simulink model "Delta_Sigma_ADC_Deg3"  (R2025b)
settings: Solver=VariableStepAuto  StartTime=0.0  StopTime=15  RelTol=1e-3
undefined symbols (not defined in the file): DiscIntNeverNeededParam
settings Model: Creator=Yash  LastModifiedBy=Yash
settings DataIOCC: SaveOutput=off  SaveTime=off
settings HardwareCC: ProdBitPerPointer=32.0  ProdBitPerSizeT=32.0  ProdBitPerPtrDiffT=32.0  ProdLargestAtomicFloat=None  ProdIntDivRoundTo=Undefined  ProdEndianess=Unspecified  ProdWordSize=32.0  ProdHWDeviceType=ASIC/FPGA->ASIC/FPGA  TargetBitPerPointer=64.0  TargetBitPerSizeT=64.0  TargetBitPerPtrDiffT=64.0  TargetLongLongMode=on  TargetIntDivRoundTo=Zero  TargetEndianess=LittleEndian  TargetWordSize=64.0  TargetHWDeviceType=Custom Processor->MATLAB Host Computer  ProdEqTarget=off

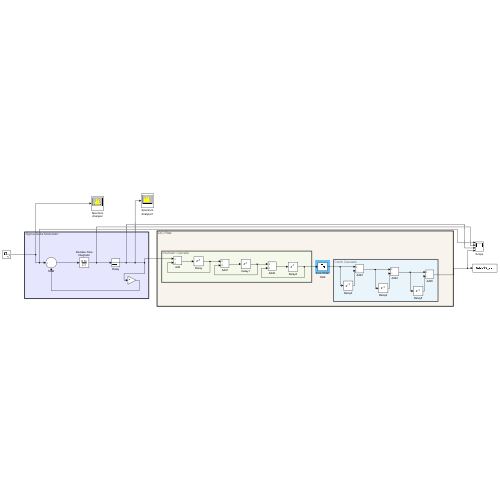
[thumbnail: Simulink's stored preview of the top-level diagram]
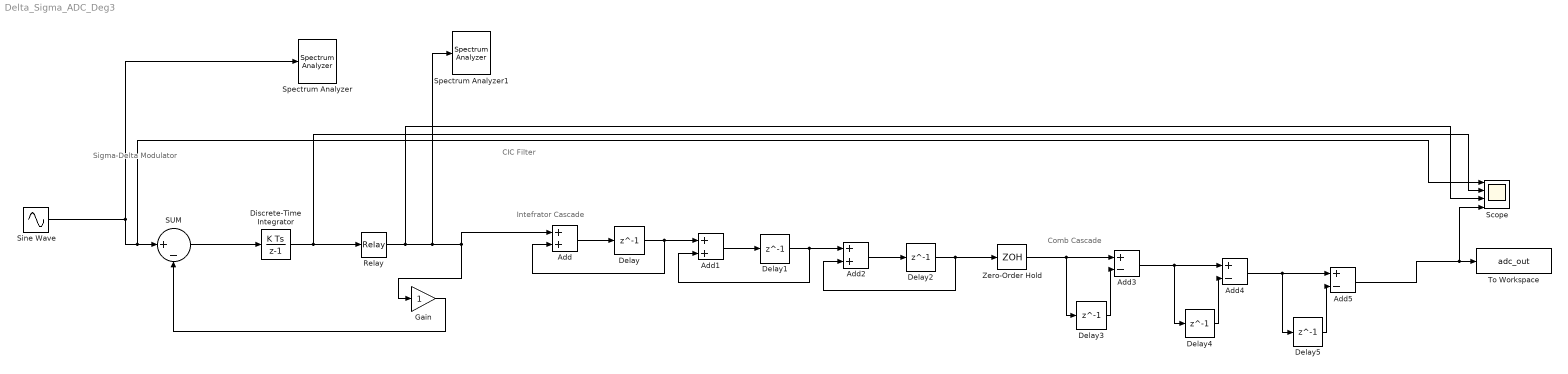
== system Delta_Sigma_ADC_Deg3 ==
  note: CIC Filter
  note: Comb Cascade
  note: Intefrator Cascade
  note: Sigma-Delta Modulator
  Add : Sum
  Add1 : Sum
  Add2 : Sum
  Add3 : Sum  Inputs=+-
  Add4 : Sum  Inputs=+-
  Add5 : Sum  Inputs=+-
  Delay{,1..5} (6 alike) : Delay  DelayLength=1
  Discrete-Time Integrator : DiscreteIntegrator  SampleTime=1/128000  ICPrevOutput=DiscIntNeverNeededParam  ICPrevScaledInput=DiscIntNeverNeededParam
  Gain : Gain
  Relay : Relay  OnSwitchValue=0  OffSwitchValue=0  OffOutputValue=-1
  SUM : Sum  Inputs=|+-
  Scope : Scope  NumInputPorts=4
      settings: ActiveDisplayYMinimum=-0.87499999999381883  ActiveDisplayYMaximum=0.87499999999757749
  Sine Wave : Sin  Amplitude=0.7  SampleTime=1/128000
  Spectrum Analyzer : SpectrumAnalyzer  WindowPosition=[2.000000,50.000000,766.000000,377.000000,]  Visible=on  ScopeFrameLocation=window  Method=Welch  PlotAsTwoSidedSpectrum=off  FrequencyScale=Log  AveragingMethod=Exponential  YLimits=[-345.0297 59.0473]  SelectedToolstripTab=spectrumAnalyzerToolstrip.spectrumTab
  Spectrum Analyzer1 : SpectrumAnalyzer  WindowPosition=[770.000000,50.000000,766.000000,377.000000,]  Visible=on  ScopeFrameLocation=window  Method=Welch  PlotAsTwoSidedSpectrum=off  FrequencyScale=Log  AveragingMethod=Exponential  MaximizeAxes=Off  YLimits=[-58.9779 27.2634]  SelectedToolstripTab=spectrumAnalyzerToolstrip.channelMeasurementsTab
  To Workspace : ToWorkspace  VariableName=adc_out  SampleTime=-1
  Zero-Order Hold : ZeroOrderHold  SampleTime=256/128000
  wires:
  SUM/1 -> Discrete-Time Integrator/1
  Discrete-Time Integrator/1 -> Scope/2, Relay/1
  Gain/1 -> SUM/2
  Sine Wave/1 -> Scope/1, SUM/1, Spectrum Analyzer/1
  Add/1 -> Delay/1
  Delay/1 -> Add1/1, Add/2
  Delay1/1 -> Add2/1, Add1/2
  Add1/1 -> Delay1/1
  Delay2/1 -> Zero-Order Hold/1, Add2/2
  Add2/1 -> Delay2/1
  Zero-Order Hold/1 -> Delay3/1, Add3/1
  Delay3/1 -> Add3/2
  Delay4/1 -> Add4/2
  Add3/1 -> Delay4/1, Add4/1
  Delay5/1 -> Add5/2
  Add4/1 -> Delay5/1, Add5/1
  Relay/1 -> Scope/3, Gain/1, Add/1, Spectrum Analyzer1/1
  Add5/1 -> Scope/4, To Workspace/1
